simulink model "MotorCD"  (R2020b)
settings: Solver=VariableStepAuto  StartTime=0.0  StopTime=10.0  RelTol=1e-3
libraries: cstblocks x2
settings Model: Creator=segamboa  LastModifiedBy=segamboa

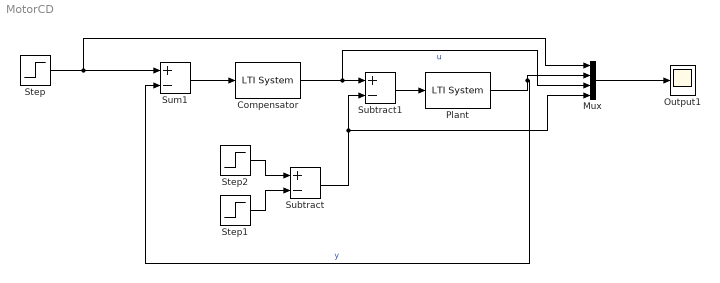
== system MotorCD ==
  Compensator : cstblocks/LTI System  sys=C  IC=[]
  Mux : Mux
  Output1 : Scope
  Plant : cstblocks/LTI System  sys=G  IC=[]
  Step : Step  Time=0.1  After=4  SampleTime=0
  Step1 : Step  Time=1.2  SampleTime=0
  Step2 : Step  Time=0.7  SampleTime=0
  Subtract : Sum  Inputs=+-
  Subtract1 : Sum  Inputs=+-
  Sum1 : Sum  Inputs=+-
  wires:
  Step/1 -> Mux/1, Sum1/1
  Mux/1 -> Output1/1
  Step1/1 -> Subtract/2
  Step2/1 -> Subtract/1
  Subtract1/1 -> Plant/1
  Plant/1 -> Mux/2, Sum1/2  "y"
  Sum1/1 -> Compensator/1
  Subtract/1 -> Mux/4, Subtract1/2
  Compensator/1 -> Mux/3, Subtract1/1  "u"
